simulink model "afs"  (R2024a)
settings: Solver=VariableStepAuto  StartTime=0.0  StopTime=5  RelTol=1e-3
libraries: simulink x1
settings Model: Creator=cheba  LastModifiedBy=cheba

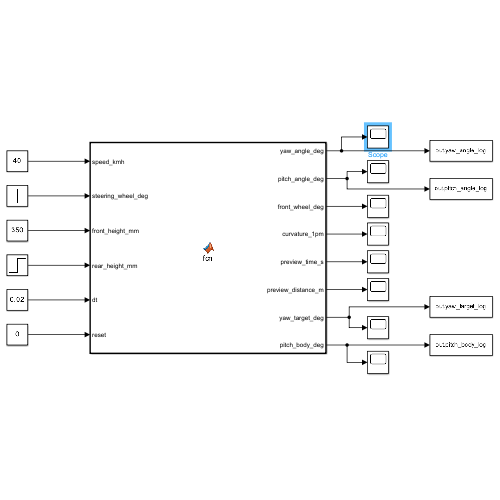
[thumbnail: Simulink's stored preview of the top-level diagram]
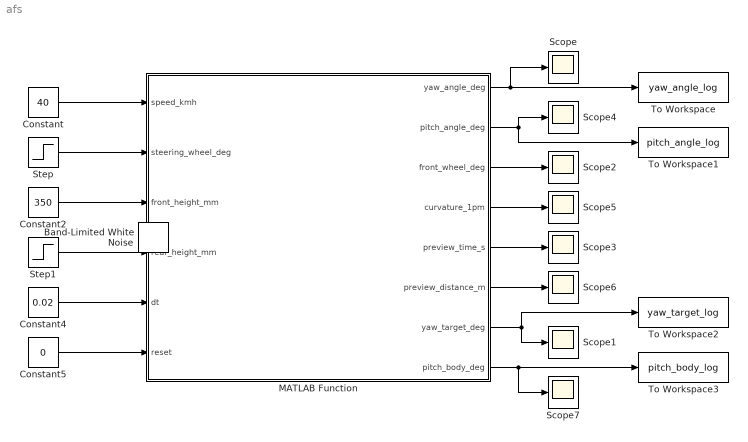
== system afs ==
  Constant : Constant  Value=40
  Constant2 : Constant  Value=350
  Constant4 : Constant  Value=0.02
  Constant5 : Constant  Value=0
  MATLAB Function : MATLAB Function  TreatAsAtomicUnit=on
  Scope{,1..7} (8 alike) : Scope
  Step : Step  After=90  SampleTime=0
  Step1 : Step  Time=2  Before=350  After=370  SampleTime=0
  To Workspace : ToWorkspace  VariableName=yaw_angle_log  SaveFormat=Structure With Time  SampleTime=-1
  To Workspace1 : ToWorkspace  VariableName=pitch_angle_log  SaveFormat=Structure With Time  SampleTime=-1
  To Workspace2 : ToWorkspace  VariableName=yaw_target_log  SaveFormat=Structure With Time  SampleTime=-1
  To Workspace3 : ToWorkspace  VariableName=pitch_body_log  SaveFormat=Structure With Time  SampleTime=-1
  Band-Limited White Noise : simulink/Sources/Band-Limited White Noise  IOType=siggen  Cov=[0.1]  Ts=0.1  seed=[23341]
      settings: LibrarySourceBlock=|
      | simgens/Band-Limited
      | White Noise
  wires:
  Constant/1 -> MATLAB Function/1(speed_kmh)
  Step/1 -> MATLAB Function/2(steering_wheel_deg)
  Constant2/1 -> MATLAB Function/3(front_height_mm)
  Step1/1 -> MATLAB Function/4(rear_height_mm)
  Constant4/1 -> MATLAB Function/5(dt)
  Constant5/1 -> MATLAB Function/6(reset)
  MATLAB Function/1(yaw_angle_deg) -> Scope/1, To Workspace/1
  MATLAB Function/2(pitch_angle_deg) -> To Workspace1/1, Scope4/1
  MATLAB Function/3(front_wheel_deg) -> Scope2/1
  MATLAB Function/4(curvature_1pm) -> Scope5/1
  MATLAB Function/5(preview_time_s) -> Scope3/1
  MATLAB Function/6(preview_distance_m) -> Scope6/1
  MATLAB Function/7(yaw_target_deg) -> To Workspace2/1, Scope1/1
  MATLAB Function/8(pitch_body_deg) -> To Workspace3/1, Scope7/1

== matlab function afs/MATLAB Function ==
  data: speed_kmh input; yaw_angle_deg output; steering_wheel_deg input; front_height_mm input; rear_height_mm input; dt input; reset input; pitch_angle_deg output; front_wheel_deg output; curvature_1pm output; preview_time_s output; preview_distance_m output; yaw_target_deg output; pitch_body_deg output
function [yaw_angle_deg, pitch_angle_deg, front_wheel_deg, curvature_1pm, ...
          preview_time_s, preview_distance_m, yaw_target_deg, pitch_body_deg] = ...
          fcn(speed_kmh, steering_wheel_deg, front_height_mm, rear_height_mm, dt, reset)

[yaw_angle_deg, pitch_angle_deg, front_wheel_deg, curvature_1pm, ...
 preview_time_s, preview_distance_m, yaw_target_deg, pitch_body_deg] = ...
    afs_controller_simulink(speed_kmh, steering_wheel_deg, ...
                            front_height_mm, rear_height_mm, dt, reset);
